simulink model "Hopper_Land_Sim"  (R2023b)
settings: Solver=VariableStepAuto  StartTime=0.0  StopTime=64.5  FixedStep=0.1  MaxStep=0.1  RelTol=1e-6  AbsTol=1e-8
values from neighbouring files (symbols this model uses):
  c_l = 2*sqrt(k_l*m_leg)    [SpringModels.m]
  c_s = 2    [SpringModels.m]
  c_T = 90000    [SpringModels.m]
  C_T = 0.1    [Vehicle_Properties.m]
  g = 1.625    [CalculateLQRGains.m]    (also in IterativeLQR.m; LQR_Controller.m; Trap2D.m = param.g; Vehicle_Properties.m)
  k_l = 100000000000    [SpringModels.m]
  k_s = 500    [SpringModels.m]
  k_T = 9999999    [SpringModels.m]    (also in Vehicle_Properties.m = 0.8)
  K_x = K    [LQR_Controller.m]
  K_y = [K(1), -K(2), K(3), -K(4)]    [LQR_Controller.m]
  l = 4.2926/2    (= 2.1463)    [CalculateLQRGains.m]    (also in IterativeLQR.m; LQR_Controller.m; Vehicle_Properties.m)
  m_e = 150    [CalculateLQRGains.m]    (also in IterativeLQR.m; LQR_Controller.m; Vehicle_Properties.m)
  m_l = 803    [CalculateLQRGains.m]    (also in IterativeLQR.m; LQR_Controller.m; Vehicle_Properties.m)
  m_leg = 10    [SpringModels.m]
  m_s = 355.9/2    (= 177.95)    [SpringModels.m]
  mu_floor = .2    (= 0.2)    [SpringModels.m]
  mu_surface = 0.2    [Vehicle_Properties.m]
  n_floor = [cosd(90+floor_angle), 0, sind(90+floor_angle)]    [FloorModel.m]
  n_surface = [0; 0; 1]    [Vehicle_Properties.m]
  p_l2 = [1; 0; -.5]    [SpringModels.m]
  p_l3 = [0; -1; -.5]    [SpringModels.m]
  p_l4 = [0; 1; -.5]    [SpringModels.m]
  r_l1 = [cosd(angle_legs); 0; sind(leg_length)]    [FloorModel.m]    (also in SpringModels.m = r_l1/norm(r_l1))
  r_l2 = [-cosd(angle_legs); 0; sind(leg_length)]    [FloorModel.m]    (also in SpringModels.m = r_l2/norm(r_l2))
  r_l3 = [0; cosd(angle_legs); sind(leg_length)]    [FloorModel.m]    (also in SpringModels.m = r_l3/norm(r_l3))
  r_l4 = [0; -cosd(angle_legs); sind(leg_length)]    [FloorModel.m]    (also in SpringModels.m = r_l4/norm(r_l4))
libraries: matrix_library x17, slpidlib x5, simulink x2, simulink_extras x1, shared6dof x1, vrlib x1
(part 1 of 2)
settings Model: Creator=Hoboness  LastModifiedBy=tonie

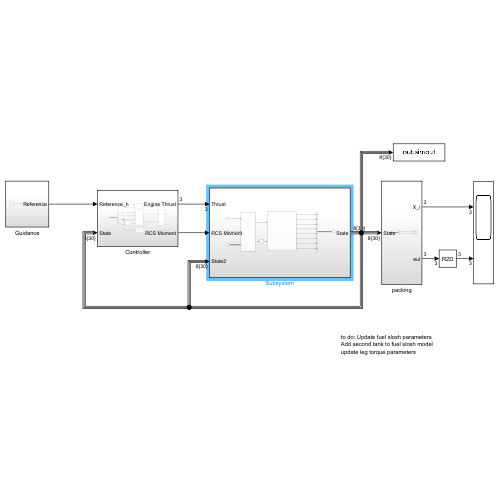
[thumbnail: Simulink's stored preview of the top-level diagram]
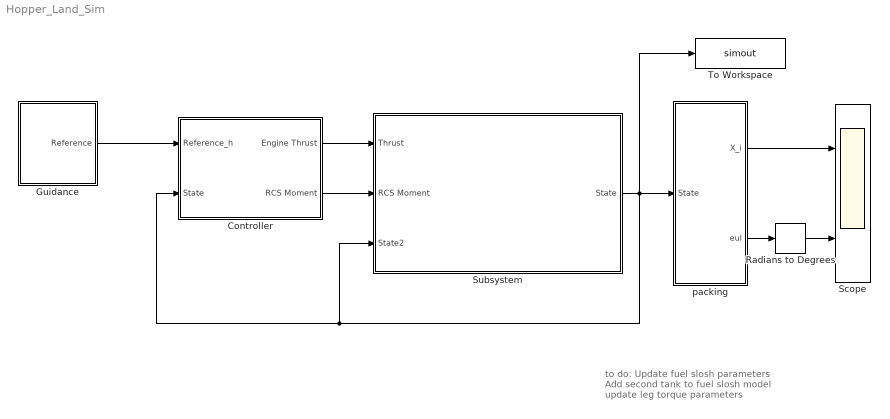
== system Hopper_Land_Sim ==
  note: to do: Update fuel slosh parameters
      | Add second tank to fuel slosh model
      | update leg torque parameters
  Controller : Subsystem
  Guidance : Subsystem
  Radians to Degrees : simulink_extras/Transformations/Radians to Degrees
  Scope : Scope  NumInputPorts=2
  Subsystem : Subsystem
  To Workspace : ToWorkspace  VariableName=simout  SaveFormat=Timeseries  SampleTime=-1
  packing : Subsystem
  wires:
  Subsystem/1(State) -> Subsystem/3(State2), Controller/2(State), packing/1(State), To Workspace/1
  Controller/1(Engine Thrust) -> Subsystem/1(Thrust)
  Guidance/1(Reference) -> Controller/1(Reference_h)
  packing/1(X_i) -> Scope/1
  packing/2(eul) -> Radians to Degrees/1
  Radians to Degrees/1 -> Scope/2
  Controller/2(RCS Moment) -> Subsystem/2(RCS Moment)

== system Hopper_Land_Sim/Controller ==
  Reference_h : Inport
  State : Inport  Port=2
  Bus Selector : BusSelector  OutputSignals=X_i,V_i,euler_a_rad,omega_b
  Psi Control : Subsystem
  Thrust Bounding : Subsystem
  X-Y control : Subsystem
  Z Control : Subsystem
  pqr to theta_dot : Subsystem
  Engine Thrust : Outport
  RCS Moment : Outport  Port=2
  wires:
  Reference_h/1 -> Z Control/1(Reference_h)
  State/1 -> Bus Selector/1
  Bus Selector/1 -> X-Y control/1(<X_i>), Z Control/2(<X_i>)  "<X_i>"
  Bus Selector/2 -> X-Y control/2(V_i)  "<V_i>"
  Bus Selector/4 -> pqr to theta_dot/2(omega_b)  "<omega_b>"
  Bus Selector/3 -> Psi Control/1(euler_a_rad), pqr to theta_dot/1(<euler_a_rad>), X-Y control/3(euler_a_rad)  "<euler_a_rad>"
  Thrust Bounding/1(Thrust) -> Engine Thrust/1
  pqr to theta_dot/1(euler_dot) -> X-Y control/4(euler_dot)
  Psi Control/1(RCS Moment) -> RCS Moment/1
  Z Control/1(Tz) -> Thrust Bounding/1(T_z)
  X-Y control/1(Tx) -> Thrust Bounding/2(Tx)
  X-Y control/2(Ty) -> Thrust Bounding/3(Ty)

== system Hopper_Land_Sim/Guidance ==
  Constant : Constant  Value=14
  Reference : Outport
  wires:
  Constant/1 -> Reference/1

== system Hopper_Land_Sim/Subsystem ==
  Thrust : Inport
  RCS Moment : Inport  Port=2
  State2 : Inport  Port=3
  6DOF (Euler Angles) : shared6dof/6DOF (Euler Angles)  units=Metric (MKS)  mtype=Fixed  rep=Euler Angles  xme_0=[0 0 100]  Vm_0=[0 0 0]  eul_0=deg2rad([0 0 0])  pm_0=[0 0 0]  mass_0=m_e + m_l  mass_e=0.5  mass_f=2.0  inertia=diag([38875.267 39854.689 26895.658]) * 0.3048^2 * 4.44822  inertia_e=eye(3)  inertia_f=2*eye(3)  k_quat=1.0  vre_flag=on  abi_flag=off  aMode=0  xme_statename=''  Vm_statename=''  eul_statename=''  quat_statename=''  pm_statename=''  mass_statename=''
  Bus Creator : BusCreator  Inputs=8
  Calculate Forces and Moments : Subsystem
  Reshape : Reshape
  State : Outport
  wires:
  6DOF (Euler Angles)/3 -> Bus Creator/3  "euler_a_rad"
  6DOF (Euler Angles)/8 -> Bus Creator/8  "A_bb"
  6DOF (Euler Angles)/4 -> Bus Creator/4  "DCM_bi"
  6DOF (Euler Angles)/6 -> Bus Creator/6  "omega_b"
  6DOF (Euler Angles)/7 -> Bus Creator/7  "omega_dot_b"
  6DOF (Euler Angles)/2 -> Bus Creator/2  "X_i"
  Bus Creator/1 -> State/1  "State"
  6DOF (Euler Angles)/1 -> Bus Creator/1  "V_i"
  6DOF (Euler Angles)/5 -> Bus Creator/5  "V_b"
  Thrust/1 -> Calculate Forces and Moments/1(Thrust)
  Calculate Forces and Moments/1(F_b) -> 6DOF (Euler Angles)/1
  Calculate Forces and Moments/2(M_b) -> Reshape/1
  State2/1 -> Calculate Forces and Moments/3(State2)
  RCS Moment/1 -> Calculate Forces and Moments/2(RCS Moment)
  Reshape/1 -> 6DOF (Euler Angles)/2

== system Hopper_Land_Sim/packing ==
  State : Inport
  Bus Selector : BusSelector  OutputSignals=X_i,euler_a_rad
  X_i : Outport
  eul : Outport  Port=2
  wires:
  State/1 -> Bus Selector/1
  Bus Selector/1 -> X_i/1  "<X_i>"
  Bus Selector/2 -> eul/1  "<euler_a_rad>"

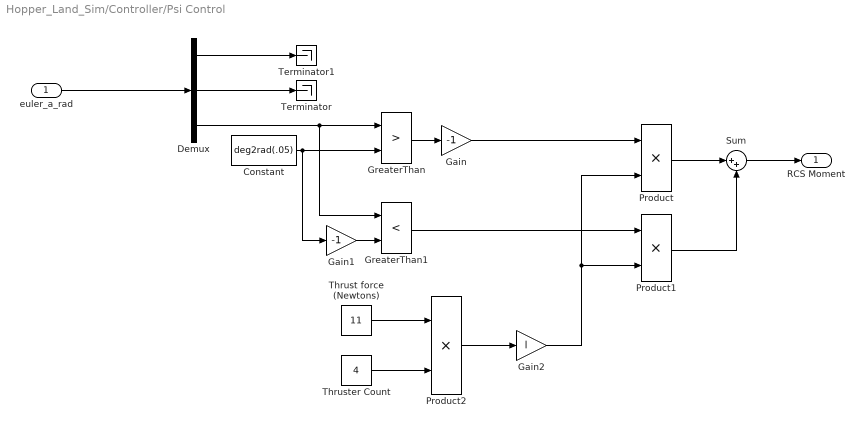
== system Hopper_Land_Sim/Controller/Psi Control ==
  euler_a_rad : Inport
  Constant : Constant  Value=deg2rad(.05)
  Demux : Demux  Outputs=3
  Gain : Gain  Gain=-1
  Gain1 : Gain  Gain=-1
  Gain2 : Gain  Gain=l
  GreaterThan : RelationalOperator  Operator=>  OutDataTypeStr=boolean  RndMeth=Simplest  InputSameDT=off
  GreaterThan1 : RelationalOperator  Operator=<  OutDataTypeStr=boolean  RndMeth=Simplest  InputSameDT=off
  Product : Product
  Product1 : Product
  Product2 : Product
  Sum : Sum  Inputs=|++
  Terminator : Terminator
  Terminator1 : Terminator
  Thrust force (Newtons) : Constant  Value=11
  Thruster Count : Constant  Value=4
  RCS Moment : Outport
  wires:
  euler_a_rad/1 -> Demux/1
  Demux/3 -> GreaterThan1/1, GreaterThan/1
  Demux/2 -> Terminator/1
  Demux/1 -> Terminator1/1
  Constant/1 -> GreaterThan/2, Gain1/1
  GreaterThan/1 -> Gain/1
  Gain/1 -> Product/1
  Product/1 -> Sum/1
  Gain1/1 -> GreaterThan1/2
  GreaterThan1/1 -> Product1/1
  Product1/1 -> Sum/2
  Thrust force (Newtons)/1 -> Product2/1
  Thruster Count/1 -> Product2/2
  Product2/1 -> Gain2/1
  Sum/1 -> RCS Moment/1
  Gain2/1 -> Product/2, Product1/2

== system Hopper_Land_Sim/Controller/Thrust Bounding ==
  T_z : Inport
  Tx : Inport  Port=2
  Ty : Inport  Port=3
  Vector Concatenate : Concatenate  NumInputs=3
  Thrust : Outport
  wires:
  T_z/1 -> Vector Concatenate/3
  Vector Concatenate/1 -> Thrust/1
  Ty/1 -> Vector Concatenate/2
  Tx/1 -> Vector Concatenate/1

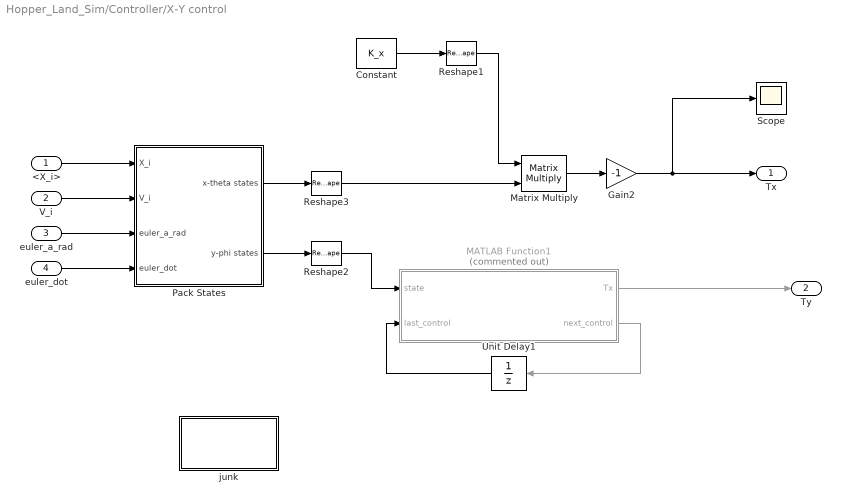
== system Hopper_Land_Sim/Controller/X-Y control ==
  <X_i> : Inport
  V_i : Inport  Port=2
  euler_a_rad : Inport  Port=3
  euler_dot : Inport  Port=4
  Constant : Constant  Value=K_x
  Gain2 : Gain  Gain=-1
  MATLAB Function1 : MATLAB Function  Commented=on  TreatAsAtomicUnit=on
  Matrix Multiply : Product  Multiplication=Matrix(*)
  "Pack States " : Subsystem
  Reshape1 : Reshape  OutputDimensionality=Row vector (2-D)
  Reshape2 : Reshape  OutputDimensionality=Column vector (2-D)
  Reshape3 : Reshape  OutputDimensionality=Column vector (2-D)
  Scope : Scope
  Unit Delay1 : UnitDelay  SampleTime=-1  HasFrameUpgradeWarning=on
  junk : Subsystem
  Tx : Outport
  Ty : Outport  Port=2
  wires:
  <X_i>/1 -> "Pack States "/1(X_i)
  V_i/1 -> "Pack States "/2(V_i)
  euler_a_rad/1 -> "Pack States "/3(euler_a_rad)
  euler_dot/1 -> "Pack States "/4(euler_dot)
  "Pack States "/2(y-phi states) -> Reshape2/1
  "Pack States "/1(x-theta states) -> Reshape3/1
  MATLAB Function1/1(Tx) -> Ty/1
  MATLAB Function1/2(next_control) -> Unit Delay1/1
  Unit Delay1/1 -> MATLAB Function1/2(last_control)
  Reshape2/1 -> MATLAB Function1/1(state)
  Gain2/1 -> Scope/1, Tx/1
  Constant/1 -> Reshape1/1
  Matrix Multiply/1 -> Gain2/1
  Reshape1/1 -> Matrix Multiply/1
  Reshape3/1 -> Matrix Multiply/2

== system Hopper_Land_Sim/Controller/Z Control ==
  Reference_h : Inport
  <X_i> : Inport  Port=2
  PID Controller : slpidlib/PID Controller  Controller=PID  Form=Parallel  TimeDomain=Continuous-time  UseExternalTs=off  SampleTime=-1  IntegratorMethod=Forward Euler  FilterMethod=Forward Euler  ControllerParametersSource=internal  P=522.596849697367  I=13.9356720912904  UseKiTs=off  D=12000  N=1  UseFilter=on  TunerSelectOption=Transfer Function Based (PID Tuner App)  InitialConditionSource=internal  InitialConditionForIntegrator=100  InitialConditionForFilter=100  DifferentiatorICPrevScaledInput=0  ExternalReset=none  TrackingMode=off  Kt=1  LimitOutput=on  SatLimitsSource=internal  UpperSaturationLimit=24000  LowerSaturationLimit=100  LinearizeAsGain=on  AntiWindupMode=none  Kb=1  LimitIntegrator=off  UpperIntegratorSaturationLimit=inf  LowerIntegratorSaturationLimit=-inf  POutMin=[]  POutMax=[]  IOutMin=[]  IOutMax=[]  DOutMin=[]  DOutMax=[]  NOutMin=[]  NOutMax=[]  SumOutMin=[]  SumOutMax=[]  SaturationOutMin=[]  SaturationOutMax=[]  PParamMin=[]  PParamMax=[]  IParamMin=[]  IParamMax=[]  DParamMin=[]  DParamMax=[]  NParamMin=[]  NParamMax=[]  KbParamMin=[]  KbParamMax=[]  KtParamMin=[]  KtParamMax=[]  KbOutMin=[]  KbOutMax=[]  KtOutMin=[]  KtOutMax=[]  IntegratorOutMin=[]  IntegratorOutMax=[]  FilterOutMin=[]  FilterOutMax=[]  SumI1OutMin=[]  SumI1OutMax=[]  SumI2OutMin=[]  SumI2OutMax=[]  SumI3OutMin=[]  SumI3OutMax=[]  SumI4OutMin=[]  SumI4OutMax=[]  SumDOutMin=[]  SumDOutMax=[]  DifferentiatorOutMin=[]  DifferentiatorOutMax=[]  FilterDiffOutCoefMin=[]  FilterDiffOutCoefMax=[]  ReciprocalOutMin=[]  ReciprocalOutMax=[]  SumDenOutMin=[]  SumDenOutMax=[]  SumNumOutMin=[]  SumNumOutMax=[]  DivideOutMin=[]  DivideOutMax=[]  UdiffTsProdOutMin=[]  UdiffTsProdOutMax=[]  NTsProdOutMin=[]  NTsProdOutMax=[]  UintegralTsProdOutMin=[]  UintegralTsProdOutMax=[]  UngainTsProdOutMin=[]  UngainTsProdOutMax=[]  ClampingZeroOutDataTypeStr=Inherit: Inherit via back propagation  ClampingZeroOutMin=[]  ClampingZeroOutMax=[]  FilterDenConstantOutDataTypeStr=Inherit: Inherit via back propagation  FilterDenConstantOutMin=[]  FilterDenConstantOutMax=[]  PCopyOutDataTypeStr=Inherit: Inherit via back propagation  PCopyOutMin=[]  PCopyOutMax=[]  NCopyOutDataTypeStr=Inherit: Inherit via back propagation  NCopyOutMin=[]  NCopyOutMax=[]  IntegratorContinuousStateAttributes=''  IntegratorStateMustResolveToSignalObject=off  IntegratorRTWStateStorageClass=Auto  FilterContinuousStateAttributes=''  FilterStateMustResolveToSignalObject=off  FilterRTWStateStorageClass=Auto  ParallelPVariant=InternalParameters  IdealPVariant=Disabled  IVariant=InternalParameters  DVariant=InternalParameters  IntegratorVariant=Continuous  SatVariant=Enabled  AWVariant=Passthrough  PCopyVariant=Disabled  TRVariant=Disabled  FdbkBlocksVariant=Forward  IdealPFdbkVariant=Disabled  SatFdbkVariant=Disabled  DerivativeFilterVariant=ContFilter  NVariant=InternalParameters  NCopyVariant=Disabled  FilterICVariant=InternalICsFilter  IntegratorICVariant=InternalICs  ExternalResetVariant=Disabled  TRSumVariant=Passthrough  SumFdbkVariant=Disabled  SumVariant=Sum_PID  TsampFilterVariant=InternalTs  TsampNgainVariant=Passthrough  TsampIntegralVariant=Disabled_SignalSpec  ExternalSaturationOutDataTypeStr=Inherit: Same as second input
  Selector : Selector  InputPortWidth=3  IndexOptions=Index vector (dialog)  Indices=3  OutputSizes=1
  Sum : Sum  Inputs=+-|
  Tz : Outport
  wires:
  Reference_h/1 -> Sum/1
  Sum/1 -> PID Controller/1
  Selector/1 -> Sum/2  "alt_m"
  PID Controller/1 -> Tz/1  "T_z"
  <X_i>/1 -> Selector/1

== system Hopper_Land_Sim/Controller/pqr to theta_dot ==
  <euler_a_rad> : Inport
  omega_b : Inport  Port=2
  MATLAB Function : MATLAB Function  TreatAsAtomicUnit=on
  euler_dot : Outport
  wires:
  omega_b/1 -> MATLAB Function/2(omega_b)
  <euler_a_rad>/1 -> MATLAB Function/1(euler_a_rad)
  MATLAB Function/1(euler_dot) -> euler_dot/1

== system Hopper_Land_Sim/Subsystem/Calculate Forces and Moments ==
  Thrust : Inport
  RCS Moment : Inport  Port=2
  State2 : Inport  Port=3
  Disturbances : Subsystem
  Ground : Subsystem
  Sum Forces : Subsystem
  Sum Moments : Subsystem
  F_b : Outport
  M_b : Outport  Port=2
  wires:
  Thrust/1 -> Disturbances/1(Thurst), Sum Moments/1(Thrust), Sum Forces/1(Thrust)
  State2/1 -> Ground/1(State2), Sum Forces/3(state)
  Sum Forces/1(Force_out) -> F_b/1
  Sum Moments/1(M_b) -> M_b/1
  RCS Moment/1 -> Sum Moments/2(RCS Moment)
  Disturbances/1(Disturbance Force) -> Sum Forces/2(Disturbance Forces)
  Disturbances/2(Disturbance Moment) -> Sum Moments/3(Disturbance Moments)
  Ground/1(Ground Force) -> Sum Forces/4(Ground Force)
  Ground/2(Ground Moments) -> Sum Moments/4(Ground Moments)

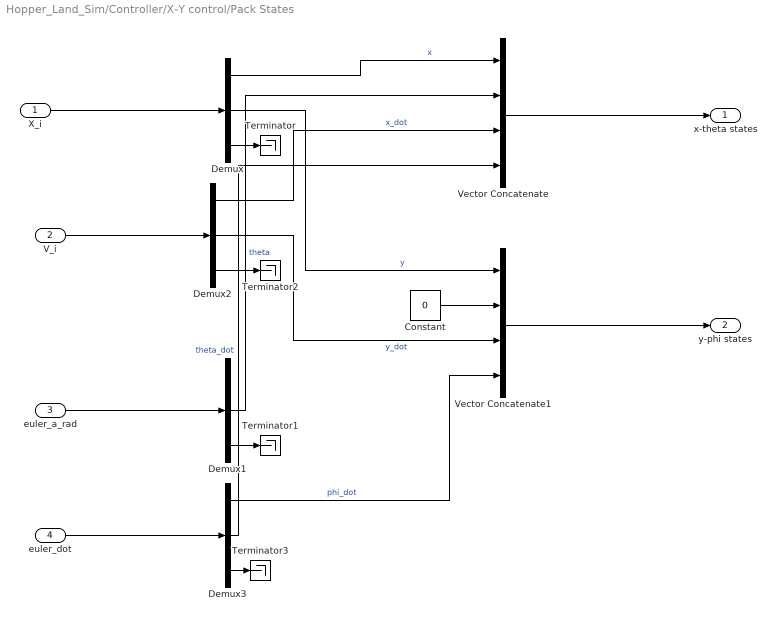
== system Hopper_Land_Sim/Controller/X-Y control/Pack States  ==
  X_i : Inport
  V_i : Inport  Port=2
  euler_a_rad : Inport  Port=3
  euler_dot : Inport  Port=4
  Constant : Constant  Value=0
  Demux{,1..3} (4 alike) : Demux  Outputs=3
  Terminator{,1..3} (4 alike) : Terminator
  Vector Concatenate : Concatenate  NumInputs=4
  Vector Concatenate1 : Concatenate  NumInputs=4
  x-theta states : Outport
  y-phi states : Outport  Port=2
  wires:
  Demux2/2 -> Vector Concatenate1/3  "y_dot"
  Demux/1 -> Vector Concatenate/1  "x"
  Demux2/1 -> Vector Concatenate/3  "x_dot"
  V_i/1 -> Demux2/1
  Demux1/3 -> Terminator1/1
  Demux/2 -> Vector Concatenate1/1  "y"
  Demux2/3 -> Terminator2/1
  Demux/3 -> Terminator/1
  Demux3/3 -> Terminator3/1
  Vector Concatenate/1 -> x-theta states/1
  X_i/1 -> Demux/1
  euler_a_rad/1 -> Demux1/1
  euler_dot/1 -> Demux3/1
  Vector Concatenate1/1 -> y-phi states/1
  Demux3/1 -> Vector Concatenate1/4  "phi_dot"
  Demux1/2 -> Vector Concatenate/2  "theta"
  Demux3/2 -> Vector Concatenate/4  "theta_dot"
  Constant/1 -> Vector Concatenate1/2

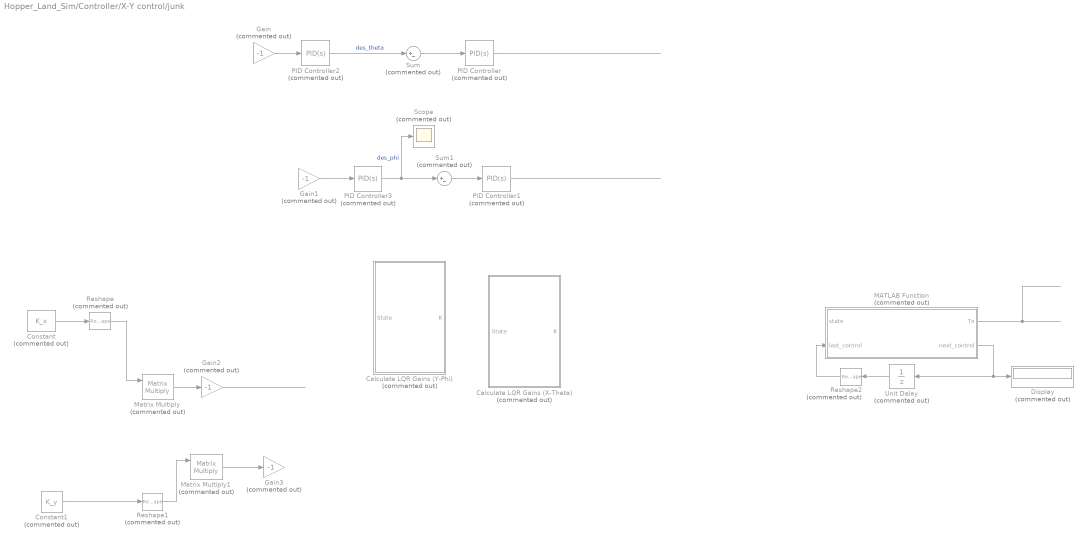
== system Hopper_Land_Sim/Controller/X-Y control/junk ==
  Calculate LQR Gains (X-Theta) : MATLAB Function  Commented=on  TreatAsAtomicUnit=on  SystemSampleTime=9999999999999
  Calculate LQR Gains (Y-Phi) : MATLAB Function  Commented=on  TreatAsAtomicUnit=on  SystemSampleTime=9999999999999
  Constant : Constant  Commented=on  Value=K_x
  Constant1 : Constant  Commented=on  Value=K_y
  Display : Display  Commented=on
  Gain{,1..3} (4 alike) : Gain  Commented=on  Gain=-1
  MATLAB Function : MATLAB Function  Commented=on  TreatAsAtomicUnit=on
  Matrix Multiply : Product  Commented=on  Multiplication=Matrix(*)
  Matrix Multiply1 : Product  Commented=on  Multiplication=Matrix(*)
  PID Controller : slpidlib/PID Controller  Commented=on  Controller=PID  Form=Parallel  TimeDomain=Continuous-time  UseExternalTs=off  SampleTime=-1  IntegratorMethod=Forward Euler  FilterMethod=Forward Euler  ControllerParametersSource=internal  P=43430.8852214789  I=11554.268575592  UseKiTs=off  D=39980.5566743985  N=32.1920872149426  UseFilter=on  TunerSelectOption=Transfer Function Based (PID Tuner App)  InitialConditionSource=internal  InitialConditionForIntegrator=0  InitialConditionForFilter=0  DifferentiatorICPrevScaledInput=0  ExternalReset=none  TrackingMode=off  Kt=1  LimitOutput=off  SatLimitsSource=internal  UpperSaturationLimit=inf  LowerSaturationLimit=-inf  LinearizeAsGain=on  AntiWindupMode=none  Kb=1  LimitIntegrator=off  UpperIntegratorSaturationLimit=inf  LowerIntegratorSaturationLimit=-inf  POutMin=[]  POutMax=[]  IOutMin=[]  IOutMax=[]  DOutMin=[]  DOutMax=[]  NOutMin=[]  NOutMax=[]  SumOutMin=[]  SumOutMax=[]  SaturationOutMin=[]  SaturationOutMax=[]  PParamMin=[]  PParamMax=[]  IParamMin=[]  IParamMax=[]  DParamMin=[]  DParamMax=[]  NParamMin=[]  NParamMax=[]  KbParamMin=[]  KbParamMax=[]  KtParamMin=[]  KtParamMax=[]  KbOutMin=[]  KbOutMax=[]  KtOutMin=[]  KtOutMax=[]  IntegratorOutMin=[]  IntegratorOutMax=[]  FilterOutMin=[]  FilterOutMax=[]  SumI1OutMin=[]  SumI1OutMax=[]  SumI2OutMin=[]  SumI2OutMax=[]  SumI3OutMin=[]  SumI3OutMax=[]  SumI4OutMin=[]  SumI4OutMax=[]  SumDOutMin=[]  SumDOutMax=[]  DifferentiatorOutMin=[]  DifferentiatorOutMax=[]  FilterDiffOutCoefMin=[]  FilterDiffOutCoefMax=[]  ReciprocalOutMin=[]  ReciprocalOutMax=[]  SumDenOutMin=[]  SumDenOutMax=[]  SumNumOutMin=[]  SumNumOutMax=[]  DivideOutMin=[]  DivideOutMax=[]  UdiffTsProdOutMin=[]  UdiffTsProdOutMax=[]  NTsProdOutMin=[]  NTsProdOutMax=[]  UintegralTsProdOutMin=[]  UintegralTsProdOutMax=[]  UngainTsProdOutMin=[]  UngainTsProdOutMax=[]  ClampingZeroOutDataTypeStr=Inherit: Inherit via back propagation  ClampingZeroOutMin=[]  ClampingZeroOutMax=[]  FilterDenConstantOutDataTypeStr=Inherit: Inherit via back propagation  FilterDenConstantOutMin=[]  FilterDenConstantOutMax=[]  PCopyOutDataTypeStr=Inherit: Inherit via back propagation  PCopyOutMin=[]  PCopyOutMax=[]  NCopyOutDataTypeStr=Inherit: Inherit via back propagation  NCopyOutMin=[]  NCopyOutMax=[]  IntegratorContinuousStateAttributes=''  IntegratorStateMustResolveToSignalObject=off  IntegratorRTWStateStorageClass=Auto  FilterContinuousStateAttributes=''  FilterStateMustResolveToSignalObject=off  FilterRTWStateStorageClass=Auto  ParallelPVariant=InternalParameters  IdealPVariant=Disabled  IVariant=InternalParameters  DVariant=InternalParameters  IntegratorVariant=Continuous  SatVariant=Disabled  AWVariant=Passthrough  PCopyVariant=Disabled  TRVariant=Disabled  FdbkBlocksVariant=Forward  IdealPFdbkVariant=Disabled  SatFdbkVariant=Disabled  DerivativeFilterVariant=ContFilter  NVariant=InternalParameters  NCopyVariant=Disabled  FilterICVariant=InternalICsFilter  IntegratorICVariant=InternalICs  ExternalResetVariant=Disabled  TRSumVariant=Passthrough  SumFdbkVariant=Disabled  SumVariant=Sum_PID  TsampFilterVariant=InternalTs  TsampNgainVariant=Passthrough  TsampIntegralVariant=Disabled_SignalSpec  ExternalSaturationOutDataTypeStr=Inherit: Same as second input
  PID Controller1 : slpidlib/PID Controller  Commented=on  Controller=PID  Form=Parallel  TimeDomain=Continuous-time  UseExternalTs=off  SampleTime=-1  IntegratorMethod=Forward Euler  FilterMethod=Forward Euler  ControllerParametersSource=internal  P=43430.8852214789  I=11554.268575592  UseKiTs=off  D=39980.5566743985  N=32.1920872149426  UseFilter=on  TunerSelectOption=Transfer Function Based (PID Tuner App)  InitialConditionSource=internal  InitialConditionForIntegrator=0  InitialConditionForFilter=0  DifferentiatorICPrevScaledInput=0  ExternalReset=none  TrackingMode=off  Kt=1  LimitOutput=off  SatLimitsSource=internal  UpperSaturationLimit=inf  LowerSaturationLimit=-inf  LinearizeAsGain=on  AntiWindupMode=none  Kb=1  LimitIntegrator=off  UpperIntegratorSaturationLimit=inf  LowerIntegratorSaturationLimit=-inf  POutMin=[]  POutMax=[]  IOutMin=[]  IOutMax=[]  DOutMin=[]  DOutMax=[]  NOutMin=[]  NOutMax=[]  SumOutMin=[]  SumOutMax=[]  SaturationOutMin=[]  SaturationOutMax=[]  PParamMin=[]  PParamMax=[]  IParamMin=[]  IParamMax=[]  DParamMin=[]  DParamMax=[]  NParamMin=[]  NParamMax=[]  KbParamMin=[]  KbParamMax=[]  KtParamMin=[]  KtParamMax=[]  KbOutMin=[]  KbOutMax=[]  KtOutMin=[]  KtOutMax=[]  IntegratorOutMin=[]  IntegratorOutMax=[]  FilterOutMin=[]  FilterOutMax=[]  SumI1OutMin=[]  SumI1OutMax=[]  SumI2OutMin=[]  SumI2OutMax=[]  SumI3OutMin=[]  SumI3OutMax=[]  SumI4OutMin=[]  SumI4OutMax=[]  SumDOutMin=[]  SumDOutMax=[]  DifferentiatorOutMin=[]  DifferentiatorOutMax=[]  FilterDiffOutCoefMin=[]  FilterDiffOutCoefMax=[]  ReciprocalOutMin=[]  ReciprocalOutMax=[]  SumDenOutMin=[]  SumDenOutMax=[]  SumNumOutMin=[]  SumNumOutMax=[]  DivideOutMin=[]  DivideOutMax=[]  UdiffTsProdOutMin=[]  UdiffTsProdOutMax=[]  NTsProdOutMin=[]  NTsProdOutMax=[]  UintegralTsProdOutMin=[]  UintegralTsProdOutMax=[]  UngainTsProdOutMin=[]  UngainTsProdOutMax=[]  ClampingZeroOutDataTypeStr=Inherit: Inherit via back propagation  ClampingZeroOutMin=[]  ClampingZeroOutMax=[]  FilterDenConstantOutDataTypeStr=Inherit: Inherit via back propagation  FilterDenConstantOutMin=[]  FilterDenConstantOutMax=[]  PCopyOutDataTypeStr=Inherit: Inherit via back propagation  PCopyOutMin=[]  PCopyOutMax=[]  NCopyOutDataTypeStr=Inherit: Inherit via back propagation  NCopyOutMin=[]  NCopyOutMax=[]  IntegratorContinuousStateAttributes=''  IntegratorStateMustResolveToSignalObject=off  IntegratorRTWStateStorageClass=Auto  FilterContinuousStateAttributes=''  FilterStateMustResolveToSignalObject=off  FilterRTWStateStorageClass=Auto  ParallelPVariant=InternalParameters  IdealPVariant=Disabled  IVariant=InternalParameters  DVariant=InternalParameters  IntegratorVariant=Continuous  SatVariant=Disabled  AWVariant=Passthrough  PCopyVariant=Disabled  TRVariant=Disabled  FdbkBlocksVariant=Forward  IdealPFdbkVariant=Disabled  SatFdbkVariant=Disabled  DerivativeFilterVariant=ContFilter  NVariant=InternalParameters  NCopyVariant=Disabled  FilterICVariant=InternalICsFilter  IntegratorICVariant=InternalICs  ExternalResetVariant=Disabled  TRSumVariant=Passthrough  SumFdbkVariant=Disabled  SumVariant=Sum_PID  TsampFilterVariant=InternalTs  TsampNgainVariant=Passthrough  TsampIntegralVariant=Disabled_SignalSpec  ExternalSaturationOutDataTypeStr=Inherit: Same as second input
  PID Controller2 : slpidlib/PID Controller  Commented=on  Controller=PID  Form=Parallel  TimeDomain=Continuous-time  UseExternalTs=off  SampleTime=-1  IntegratorMethod=Forward Euler  FilterMethod=Forward Euler  ControllerParametersSource=internal  P=0.0149555658055821  I=0.00505656866824881  UseKiTs=off  D=0  N=100  UseFilter=on  TunerSelectOption=Transfer Function Based (PID Tuner App)  InitialConditionSource=internal  InitialConditionForIntegrator=0  InitialConditionForFilter=0  DifferentiatorICPrevScaledInput=0  ExternalReset=none  TrackingMode=off  Kt=1  LimitOutput=off  SatLimitsSource=internal  UpperSaturationLimit=inf  LowerSaturationLimit=-inf  LinearizeAsGain=on  AntiWindupMode=none  Kb=1  LimitIntegrator=off  UpperIntegratorSaturationLimit=inf  LowerIntegratorSaturationLimit=-inf  POutMin=[]  POutMax=[]  IOutMin=[]  IOutMax=[]  DOutMin=[]  DOutMax=[]  NOutMin=[]  NOutMax=[]  SumOutMin=[]  SumOutMax=[]  SaturationOutMin=[]  SaturationOutMax=[]  PParamMin=[]  PParamMax=[]  IParamMin=[]  IParamMax=[]  DParamMin=[]  DParamMax=[]  NParamMin=[]  NParamMax=[]  KbParamMin=[]  KbParamMax=[]  KtParamMin=[]  KtParamMax=[]  KbOutMin=[]  KbOutMax=[]  KtOutMin=[]  KtOutMax=[]  IntegratorOutMin=[]  IntegratorOutMax=[]  FilterOutMin=[]  FilterOutMax=[]  SumI1OutMin=[]  SumI1OutMax=[]  SumI2OutMin=[]  SumI2OutMax=[]  SumI3OutMin=[]  SumI3OutMax=[]  SumI4OutMin=[]  SumI4OutMax=[]  SumDOutMin=[]  SumDOutMax=[]  DifferentiatorOutMin=[]  DifferentiatorOutMax=[]  FilterDiffOutCoefMin=[]  FilterDiffOutCoefMax=[]  ReciprocalOutMin=[]  ReciprocalOutMax=[]  SumDenOutMin=[]  SumDenOutMax=[]  SumNumOutMin=[]  SumNumOutMax=[]  DivideOutMin=[]  DivideOutMax=[]  UdiffTsProdOutMin=[]  UdiffTsProdOutMax=[]  NTsProdOutMin=[]  NTsProdOutMax=[]  UintegralTsProdOutMin=[]  UintegralTsProdOutMax=[]  UngainTsProdOutMin=[]  UngainTsProdOutMax=[]  ClampingZeroOutDataTypeStr=Inherit: Inherit via back propagation  ClampingZeroOutMin=[]  ClampingZeroOutMax=[]  FilterDenConstantOutDataTypeStr=Inherit: Inherit via back propagation  FilterDenConstantOutMin=[]  FilterDenConstantOutMax=[]  PCopyOutDataTypeStr=Inherit: Inherit via back propagation  PCopyOutMin=[]  PCopyOutMax=[]  NCopyOutDataTypeStr=Inherit: Inherit via back propagation  NCopyOutMin=[]  NCopyOutMax=[]  IntegratorContinuousStateAttributes=''  IntegratorStateMustResolveToSignalObject=off  IntegratorRTWStateStorageClass=Auto  FilterContinuousStateAttributes=''  FilterStateMustResolveToSignalObject=off  FilterRTWStateStorageClass=Auto  ParallelPVariant=InternalParameters  IdealPVariant=Disabled  IVariant=InternalParameters  DVariant=InternalParameters  IntegratorVariant=Continuous  SatVariant=Disabled  AWVariant=Passthrough  PCopyVariant=Disabled  TRVariant=Disabled  FdbkBlocksVariant=Forward  IdealPFdbkVariant=Disabled  SatFdbkVariant=Disabled  DerivativeFilterVariant=ContFilter  NVariant=InternalParameters  NCopyVariant=Disabled  FilterICVariant=InternalICsFilter  IntegratorICVariant=InternalICs  ExternalResetVariant=Disabled  TRSumVariant=Passthrough  SumFdbkVariant=Disabled  SumVariant=Sum_PID  TsampFilterVariant=InternalTs  TsampNgainVariant=Passthrough  TsampIntegralVariant=Disabled_SignalSpec  ExternalSaturationOutDataTypeStr=Inherit: Same as second input
  PID Controller3 : slpidlib/PID Controller  Commented=on  Controller=PID  Form=Parallel  TimeDomain=Continuous-time  UseExternalTs=off  SampleTime=-1  IntegratorMethod=Forward Euler  FilterMethod=Forward Euler  ControllerParametersSource=internal  P=0.0149555658055821  I=0.00505656866824881  UseKiTs=off  D=0  N=100  UseFilter=on  TunerSelectOption=Transfer Function Based (PID Tuner App)  InitialConditionSource=internal  InitialConditionForIntegrator=0  InitialConditionForFilter=0  DifferentiatorICPrevScaledInput=0  ExternalReset=none  TrackingMode=off  Kt=1  LimitOutput=off  SatLimitsSource=internal  UpperSaturationLimit=inf  LowerSaturationLimit=-inf  LinearizeAsGain=on  AntiWindupMode=none  Kb=1  LimitIntegrator=off  UpperIntegratorSaturationLimit=inf  LowerIntegratorSaturationLimit=-inf  POutMin=[]  POutMax=[]  IOutMin=[]  IOutMax=[]  DOutMin=[]  DOutMax=[]  NOutMin=[]  NOutMax=[]  SumOutMin=[]  SumOutMax=[]  SaturationOutMin=[]  SaturationOutMax=[]  PParamMin=[]  PParamMax=[]  IParamMin=[]  IParamMax=[]  DParamMin=[]  DParamMax=[]  NParamMin=[]  NParamMax=[]  KbParamMin=[]  KbParamMax=[]  KtParamMin=[]  KtParamMax=[]  KbOutMin=[]  KbOutMax=[]  KtOutMin=[]  KtOutMax=[]  IntegratorOutMin=[]  IntegratorOutMax=[]  FilterOutMin=[]  FilterOutMax=[]  SumI1OutMin=[]  SumI1OutMax=[]  SumI2OutMin=[]  SumI2OutMax=[]  SumI3OutMin=[]  SumI3OutMax=[]  SumI4OutMin=[]  SumI4OutMax=[]  SumDOutMin=[]  SumDOutMax=[]  DifferentiatorOutMin=[]  DifferentiatorOutMax=[]  FilterDiffOutCoefMin=[]  FilterDiffOutCoefMax=[]  ReciprocalOutMin=[]  ReciprocalOutMax=[]  SumDenOutMin=[]  SumDenOutMax=[]  SumNumOutMin=[]  SumNumOutMax=[]  DivideOutMin=[]  DivideOutMax=[]  UdiffTsProdOutMin=[]  UdiffTsProdOutMax=[]  NTsProdOutMin=[]  NTsProdOutMax=[]  UintegralTsProdOutMin=[]  UintegralTsProdOutMax=[]  UngainTsProdOutMin=[]  UngainTsProdOutMax=[]  ClampingZeroOutDataTypeStr=Inherit: Inherit via back propagation  ClampingZeroOutMin=[]  ClampingZeroOutMax=[]  FilterDenConstantOutDataTypeStr=Inherit: Inherit via back propagation  FilterDenConstantOutMin=[]  FilterDenConstantOutMax=[]  PCopyOutDataTypeStr=Inherit: Inherit via back propagation  PCopyOutMin=[]  PCopyOutMax=[]  NCopyOutDataTypeStr=Inherit: Inherit via back propagation  NCopyOutMin=[]  NCopyOutMax=[]  IntegratorContinuousStateAttributes=''  IntegratorStateMustResolveToSignalObject=off  IntegratorRTWStateStorageClass=Auto  FilterContinuousStateAttributes=''  FilterStateMustResolveToSignalObject=off  FilterRTWStateStorageClass=Auto  ParallelPVariant=InternalParameters  IdealPVariant=Disabled  IVariant=InternalParameters  DVariant=InternalParameters  IntegratorVariant=Continuous  SatVariant=Disabled  AWVariant=Passthrough  PCopyVariant=Disabled  TRVariant=Disabled  FdbkBlocksVariant=Forward  IdealPFdbkVariant=Disabled  SatFdbkVariant=Disabled  DerivativeFilterVariant=ContFilter  NVariant=InternalParameters  NCopyVariant=Disabled  FilterICVariant=InternalICsFilter  IntegratorICVariant=InternalICs  ExternalResetVariant=Disabled  TRSumVariant=Passthrough  SumFdbkVariant=Disabled  SumVariant=Sum_PID  TsampFilterVariant=InternalTs  TsampNgainVariant=Passthrough  TsampIntegralVariant=Disabled_SignalSpec  ExternalSaturationOutDataTypeStr=Inherit: Same as second input
  Reshape : Reshape  Commented=on  OutputDimensionality=Row vector (2-D)
  Reshape1 : Reshape  Commented=on  OutputDimensionality=Row vector (2-D)
  Reshape2 : Reshape  Commented=on  OutputDimensionality=Row vector (2-D)
  Scope : Scope  Commented=on
  Sum : Sum  Commented=on  Inputs=|+-
  Sum1 : Sum  Commented=on  Inputs=|+-
  Unit Delay : UnitDelay  Commented=on  InitialCondition=zeros(1,80)  SampleTime=-1  HasFrameUpgradeWarning=on
  wires:
  PID Controller3/1 -> Scope/1, Sum1/1  "des_phi"
  PID Controller1/1 -> ?
  ? -> Gain/1  "X"
  ? -> Sum1/2
  ? -> Gain1/1
  Gain1/1 -> PID Controller3/1
  PID Controller2/1 -> Sum/1  "des_theta"
  PID Controller/1 -> ?
  Sum1/1 -> PID Controller1/1
  Sum/1 -> PID Controller/1
  ? -> Sum/2
  Gain/1 -> PID Controller2/1
  Gain2/1 -> ?
  Matrix Multiply/1 -> Gain2/1
  Matrix Multiply1/1 -> Gain3/1
  Constant/1 -> Reshape/1
  Reshape1/1 -> Matrix Multiply1/1
  Constant1/1 -> Reshape1/1
  ? -> ?
  ? -> ?
  Reshape/1 -> Matrix Multiply/1
  Reshape2/1 -> MATLAB Function/2(last_control)
  MATLAB Function/1(Tx) -> ?
  ? -> MATLAB Function/1(state)
  Unit Delay/1 -> Reshape2/1
  MATLAB Function/2(next_control) -> Display/1, Unit Delay/1

== system Hopper_Land_Sim/Subsystem/Calculate Forces and Moments/Disturbances ==
  Thurst : Inport
  Fuel Slosh : Subsystem
  Disturbance Force : Outport
  Disturbance Moment : Outport  Port=2
  wires:
  Thurst/1 -> Fuel Slosh/1(Thrust)
  Fuel Slosh/1(Disturbance Force) -> Disturbance Force/1
  Fuel Slosh/2(Disturbance Moment) -> Disturbance Moment/1

== system Hopper_Land_Sim/Subsystem/Calculate Forces and Moments/Ground ==
  State2 : Inport
  Floor Model : Subsystem
  Floor Model1 : Subsystem  Commented=on
  Leg Model : Subsystem
  Ground Force : Outport
  Ground Moments : Outport  Port=2
  wires:
  State2/1 -> Floor Model1/1(In1), Floor Model/1(In1)
  Floor Model/1(f_T) -> Leg Model/1(f_T)
  Leg Model/1(Leg Force) -> ?
  Leg Model/2(Leg Moment) -> ?
  Floor Model1/1(f_T) -> ?

== system Hopper_Land_Sim/Subsystem/Calculate Forces and Moments/Sum Forces ==
  Thrust : Inport
  Disturbance Forces : Inport  Port=2
  state : Inport  Port=3
  Ground Force : Inport  Port=4
  Add : Sum  Inputs=++++
  Fake ground : Subsystem  Commented=on
  Gravity : Subsystem
  Ground : Subsystem  Commented=on
  Force_out : Outport
  wires:
  Gravity/1(gravity) -> Add/4
  state/1 -> Gravity/1(state), Fake ground/2(state)
  Disturbance Forces/1 -> Add/2
  Add/1 -> Force_out/1
  Thrust/1 -> Add/1
  Ground Force/1 -> Add/3

== system Hopper_Land_Sim/Subsystem/Calculate Forces and Moments/Sum Moments ==
  Thrust : Inport
  RCS Moment : Inport  Port=2
  Disturbance Moments : Inport  Port=3
  Ground Moments : Inport  Port=4
  Add : Sum  Inputs=++++
  Constant : Constant  Value=[0; 0; l]
  Constant1 : Constant  Value=0
  Cross Product : matrix_library/Cross Product
  Reshape : Reshape  OutputDimensionality=Column vector (2-D)
  Reshape1 : Reshape  OutputDimensionality=Column vector (2-D)
  Vector Concatenate : Concatenate  NumInputs=3
  M_b : Outport
  wires:
  Cross Product/1 -> Reshape/1
  Thrust/1 -> Cross Product/2
  Disturbance Moments/1 -> Add/3
  Constant/1 -> Cross Product/1
  Constant1/1 -> Vector Concatenate/2, Vector Concatenate/1
  RCS Moment/1 -> Vector Concatenate/3
  Vector Concatenate/1 -> Reshape1/1
  Reshape/1 -> Add/1
  Reshape1/1 -> Add/2
  Ground Moments/1 -> Add/4
  Add/1 -> M_b/1

== system Hopper_Land_Sim/Subsystem/Calculate Forces and Moments/Disturbances/Fuel Slosh ==
  Thrust : Inport
  Fuel Spring Model : Subsystem
  Disturbance Force : Outport
  Disturbance Moment : Outport  Port=2
  wires:
  Thrust/1 -> Fuel Spring Model/1(Thrust)
  Fuel Spring Model/1(Fuel Slosh Force) -> Disturbance Force/1
  Fuel Spring Model/2(Fuel Slosh Moment) -> Disturbance Moment/1

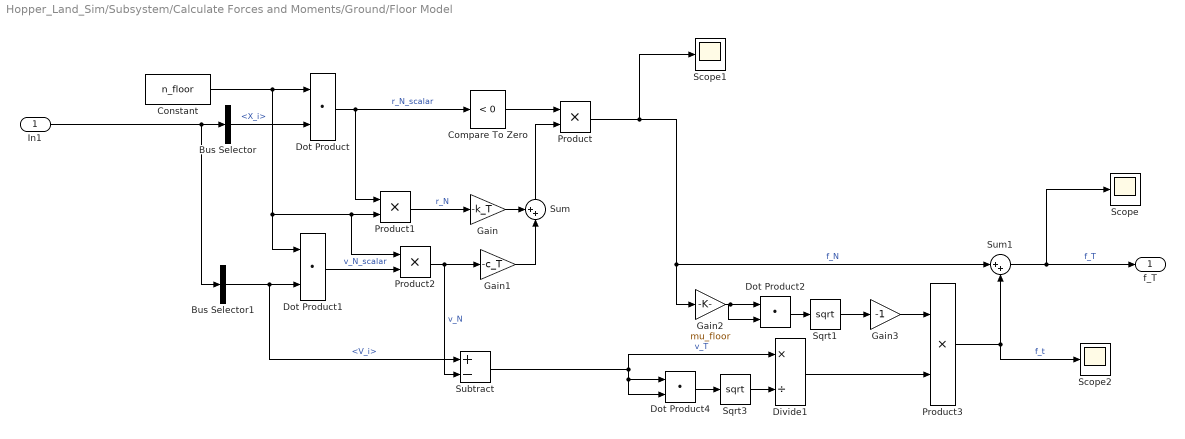
== system Hopper_Land_Sim/Subsystem/Calculate Forces and Moments/Ground/Floor Model ==
  In1 : Inport
  Bus Selector : BusSelector  OutputSignals=X_i
  Bus Selector1 : BusSelector  OutputSignals=V_i
  Compare To Zero : simulink/Logic and Bit Operations/Compare To Zero  relop=<  OutDataTypeStr=boolean
  Constant : Constant  Value=n_floor
  Divide1 : Product  Inputs=*/
  Dot Product{,1..2,4} (4 alike) : DotProduct  OutDataTypeStr=Inherit: Inherit via internal rule
  Gain : Gain  Gain=-k_T
  Gain1 : Gain  Gain=-c_T
  Gain2 : Gain  Gain=mu_floor
  Gain3 : Gain  Gain=-1
  Product{,1..3} (4 alike) : Product
  Scope : Scope
  Scope1 : Scope
  Scope2 : Scope
  Sqrt1 : Sqrt
  Sqrt3 : Sqrt
  Subtract : Sum  Inputs=+-
  Sum : Sum  Inputs=++|
  Sum1 : Sum  Inputs=|++
  f_T : Outport
  wires:
  Product2/1 -> Subtract/2, Gain1/1  "v_N"
  Bus Selector/1 -> Dot Product/2  "<X_i>"
  Constant/1 -> Dot Product1/1, Product2/1, Product1/2, Dot Product/1
  Bus Selector1/1 -> Subtract/1, Dot Product1/2  "<V_i>"
  Product3/1 -> Scope2/1, Sum1/2  "f_t"
  Dot Product1/1 -> Product2/2  "v_N_scalar"
  Product/1 -> Scope1/1, Gain2/1, Sum1/1  "f_N"
  Dot Product/1 -> Product1/1, Compare To Zero/1  "r_N_scalar"
  In1/1 -> Bus Selector1/1, Bus Selector/1
  Gain3/1 -> Product3/1
  Gain2/1 -> Dot Product2/2, Dot Product2/1
  Product1/1 -> Gain/1  "r_N"
  Sum1/1 -> f_T/1, Scope/1  "f_T"
  Dot Product2/1 -> Sqrt1/1
  Gain/1 -> Sum/1
  Sum/1 -> Product/2
  Compare To Zero/1 -> Product/1
  Gain1/1 -> Sum/2
  Sqrt1/1 -> Gain3/1
  Dot Product4/1 -> Sqrt3/1
  Divide1/1 -> Product3/2
  Sqrt3/1 -> Divide1/2
  Subtract/1 -> Divide1/1, Dot Product4/1, Dot Product4/2  "v_T"

== system Hopper_Land_Sim/Subsystem/Calculate Forces and Moments/Ground/Floor Model1 ==
  In1 : Inport
  Abs : Abs  SaturateOnIntegerOverflow=off
  Bus Selector : BusSelector  OutputSignals=X_i
  Compare To Zero : simulink/Logic and Bit Operations/Compare To Zero  relop=<  OutDataTypeStr=boolean
  Constant : Constant  Value=n_floor
  Constant1 : Constant  Value=[0; 0; 1000000]
  Dot Product : DotProduct  OutDataTypeStr=Inherit: Inherit via internal rule
  Product : Product
  f_T : Outport
  wires:
  Bus Selector/1 -> Dot Product/2  "<X_i>"
  Constant/1 -> Dot Product/1
  Dot Product/1 -> Compare To Zero/1  "r_N_scalar"
  In1/1 -> Bus Selector/1
  Compare To Zero/1 -> Product/1
  Product/1 -> Abs/1  "f_N"
  Abs/1 -> f_T/1
  Constant1/1 -> Product/2

== system Hopper_Land_Sim/Subsystem/Calculate Forces and Moments/Ground/Leg Model ==
  f_T : Inport
  Leg1 : Subsystem
  Leg2 : Subsystem
  Leg3 : Subsystem
  Leg4 : Subsystem
  Sum{1..2,5..6} (4 alike) : Sum  Inputs=++|
  Sum3 : Sum  Inputs=|++
  Sum4 : Sum  Inputs=|++
  Leg Force : Outport
  Leg Moment : Outport  Port=2
  wires:
  f_T/1 -> Leg4/1(f_T), Leg3/1(f_T), Leg2/1(f_T), Leg1/1(f_T)
  Leg3/1(f_l3) -> Sum1/1
  Leg4/1(f_l4) -> Sum1/2
  Leg2/1(f_l2) -> Sum2/1
  Sum1/1 -> Sum2/2
  ? -> Sum3/1
  Sum2/1 -> Sum3/2
  Leg1/1(m_l1) -> Sum4/1
  Leg2/2(m_l2) -> Sum5/1
  Leg3/2(m_l3) -> Sum6/1
  Leg4/2(m_l4) -> Sum6/2
  Sum6/1 -> Sum5/2
  Sum5/1 -> Sum4/2
  Sum3/1 -> Leg Force/1
  Sum4/1 -> Leg Moment/1

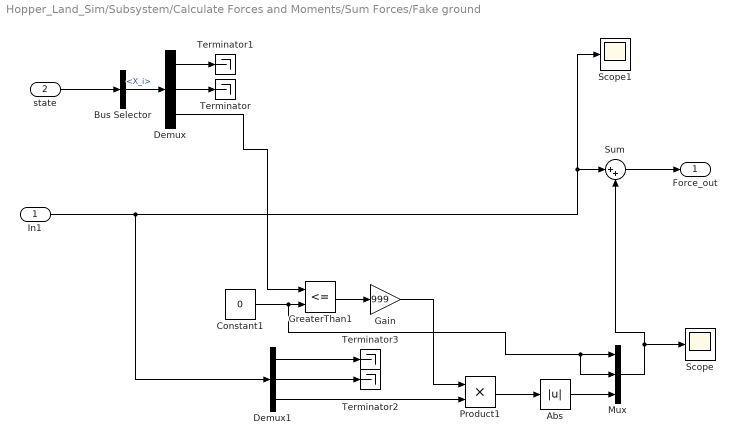
== system Hopper_Land_Sim/Subsystem/Calculate Forces and Moments/Sum Forces/Fake ground ==
  In1 : Inport
  state : Inport  Port=2
  Abs : Abs  SaturateOnIntegerOverflow=off
  Bus Selector : BusSelector  OutputSignals=X_i
  Constant1 : Constant  Value=0
  Demux : Demux  Outputs=3
  Demux1 : Demux  Outputs=3
  Gain : Gain  Gain=999
  GreaterThan1 : RelationalOperator  Operator=<=  OutDataTypeStr=boolean  RndMeth=Simplest  InputSameDT=off
  Mux : Mux  Inputs=3
  Product1 : Product
  Scope : Scope
  Scope1 : Scope
  Sum : Sum  Inputs=|++
  Terminator{,1..3} (4 alike) : Terminator
  Force_out : Outport
  wires:
  state/1 -> Bus Selector/1
  Bus Selector/1 -> Demux/1  "<X_i>"
  Demux/2 -> Terminator/1
  Demux/1 -> Terminator1/1
  Demux/3 -> GreaterThan1/1
  Constant1/1 -> Mux/2, Mux/1, GreaterThan1/2
  GreaterThan1/1 -> Gain/1
  Gain/1 -> Product1/1
  Product1/1 -> Abs/1
  Sum/1 -> Force_out/1
  In1/1 -> Demux1/1, Scope1/1, Sum/1
  Demux1/3 -> Product1/2
  Abs/1 -> Mux/3
  Demux1/2 -> Terminator2/1
  Demux1/1 -> Terminator3/1
  Mux/1 -> Sum/2, Scope/1

== system Hopper_Land_Sim/Subsystem/Calculate Forces and Moments/Sum Forces/Gravity ==
  state : Inport
  Bus Selector : BusSelector  OutputSignals=DCM_bi
  Constant1 : Constant  Value=[0; 0; -g]
  Gravity Force : Gain  Gain=m_e+m_l
  Matrix Multiply : Product  Multiplication=Matrix(*)
  gravity : Outport
  wires:
  Constant1/1 -> Matrix Multiply/2
  Gravity Force/1 -> gravity/1
  state/1 -> Bus Selector/1
  Bus Selector/1 -> Matrix Multiply/1  "<DCM_bi>"
  Matrix Multiply/1 -> Gravity Force/1

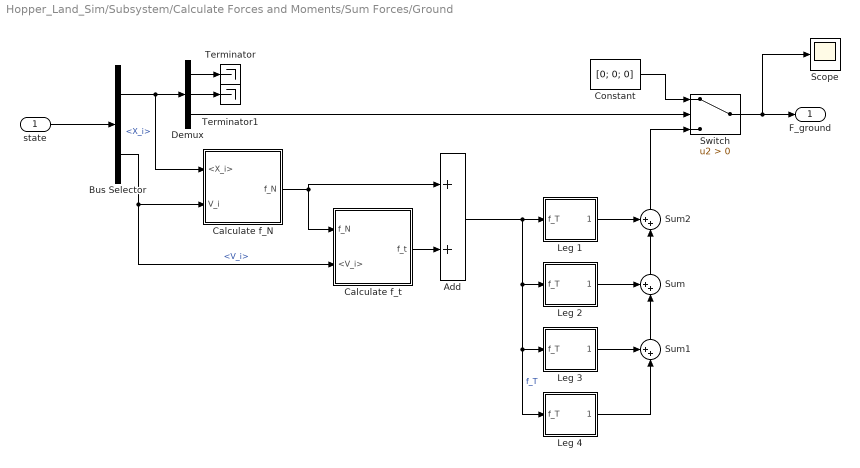
== system Hopper_Land_Sim/Subsystem/Calculate Forces and Moments/Sum Forces/Ground ==
  state : Inport
  Add : Sum
  Bus Selector : BusSelector  OutputSignals=X_i,V_i
  Calculate f_N : Subsystem
  Calculate f_t : Subsystem
  Constant : Constant  Value=[0; 0; 0]
  Demux : Demux  Outputs=3
  Leg 1 : Subsystem
  Leg 2 : Subsystem
  Leg 3 : Subsystem
  Leg 4 : Subsystem
  Scope : Scope
  Sum : Sum  Inputs=++|
  Sum1 : Sum  Inputs=++|
  Sum2 : Sum  Inputs=++|
  Switch : Switch  Criteria=u2 > Threshold  SaturateOnIntegerOverflow=off  InputSameDT=off
  Terminator : Terminator
  Terminator1 : Terminator
  F_ground : Outport
  wires:
  state/1 -> Bus Selector/1
  Bus Selector/1 -> Calculate f_N/1(<X_i>), Demux/1  "<X_i>"
  Demux/3 -> Switch/2
  Constant/1 -> Switch/1
  Switch/1 -> Scope/1, F_ground/1
  Bus Selector/2 -> Calculate f_t/2(<V_i>), Calculate f_N/2(V_i)  "<V_i>"
  Calculate f_N/1(f_N) -> Add/1, Calculate f_t/1(f_N)
  Calculate f_t/1(f_t) -> Add/2
  Add/1 -> Leg 1/1(f_T), Leg 2/1(f_T), Leg 4/1(f_T), Leg 3/1(f_T)  "f_T"
  Demux/1 -> Terminator/1
  Demux/2 -> Terminator1/1
  Leg 2/1(Outport) -> Sum/1
  Leg 3/1(Outport) -> Sum1/1
  Leg 4/1(Outport) -> Sum1/2
  Sum1/1 -> Sum/2
  Sum/1 -> Sum2/2
  Leg 1/1(Outport) -> Sum2/1
  Sum2/1 -> Switch/3

== system Hopper_Land_Sim/Subsystem/Calculate Forces and Moments/Disturbances/Fuel Slosh/Fuel Spring Model ==
  Thrust : Inport
  LOX Model : Subsystem
  Fuel Slosh Force : Outport
  Fuel Slosh Moment : Outport  Port=2
  wires:
  Thrust/1 -> LOX Model/1(Thrust)
  LOX Model/2(LOX Fuel Slosh Moment) -> Fuel Slosh Moment/1
  LOX Model/1(LOX Fuel Slosh Force) -> Fuel Slosh Force/1

== system Hopper_Land_Sim/Subsystem/Calculate Forces and Moments/Ground/Leg Model/Leg1 ==
  f_T : Inport
  Constant : Constant  Value=r_l1
  Cross Product : matrix_library/Cross Product
  Dot Product : DotProduct  OutDataTypeStr=Inherit: Inherit via internal rule
  Gain : Gain  Gain=1/m_s
  Gain1 : Gain
  Gain2 : Gain
  Integrator : Integrator
  Integrator1 : Integrator
  Product : Product
  Step : Step  Before=[0 0 100]  After=[0 0 0]  SampleTime=0
  Sum : Sum  Inputs=|++
  Sum1 : Sum  Inputs=|++
  m_l1 : Outport
  wires:
  f_T/1 -> Cross Product/1, Dot Product/1
  Constant/1 -> Cross Product/2, Product/2, Dot Product/2
  Dot Product/1 -> Product/1
  Product/1 -> ?  "f_Tt"
  ? -> m_l1/1
  Cross Product/1 -> ?  "f_Tn"
  Sum/1 -> Gain/1
  Integrator/1 -> Gain1/1, Integrator1/1  "d_dot*rhat"
  Integrator1/1 -> Gain2/1  "d"
  Sum1/1 -> Sum/2
  Step/1 -> Sum/1
  Gain/1 -> Integrator/1  "S_ddot"
  Gain1/1 -> Sum1/2
  Gain2/1 -> Sum1/1

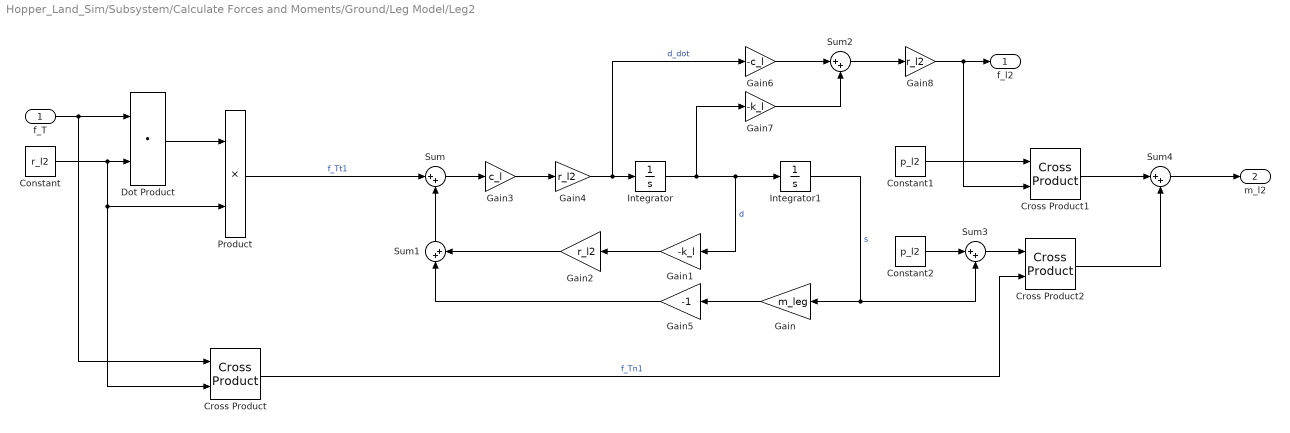
== system Hopper_Land_Sim/Subsystem/Calculate Forces and Moments/Ground/Leg Model/Leg2 ==
  f_T : Inport
  Constant : Constant  Value=r_l2
  Constant1 : Constant  Value=p_l2
  Constant2 : Constant  Value=p_l2
  Cross Product : matrix_library/Cross Product
  Cross Product1 : matrix_library/Cross Product
  Cross Product2 : matrix_library/Cross Product
  Dot Product : DotProduct  OutDataTypeStr=Inherit: Inherit via internal rule
  Gain : Gain  Gain=m_leg
  Gain1 : Gain  Gain=-k_l
  Gain2 : Gain  Gain=r_l2
  Gain3 : Gain  Gain=c_l
  Gain4 : Gain  Gain=r_l2
  Gain5 : Gain  Gain=-1
  Gain6 : Gain  Gain=-c_l
  Gain7 : Gain  Gain=-k_l
  Gain8 : Gain  Gain=r_l2
  Integrator : Integrator
  Integrator1 : Integrator
  Product : Product
  Sum{,1..4} (5 alike) : Sum  Inputs=|++
  f_l2 : Outport
  m_l2 : Outport  Port=2
  wires:
  Sum4/1 -> m_l2/1
  Cross Product2/1 -> Sum4/2
  Cross Product1/1 -> Sum4/1
  Sum3/1 -> Cross Product2/1
  Constant2/1 -> Sum3/1
  Constant1/1 -> Cross Product1/1
  Gain8/1 -> f_l2/1, Cross Product1/2
  Sum2/1 -> Gain8/1
  Gain7/1 -> Sum2/2
  Gain6/1 -> Sum2/1
  Gain5/1 -> Sum1/1
  Gain/1 -> Gain5/1
  Sum1/1 -> Sum/2
  Gain2/1 -> Sum1/2
  Sum/1 -> Gain3/1
  Gain4/1 -> Integrator/1, Gain6/1  "d_dot"
  Gain1/1 -> Gain2/1
  Integrator1/1 -> Gain/1, Sum3/2  "s"
  Integrator/1 -> Integrator1/1, Gain1/1, Gain7/1  "d"
  Gain3/1 -> Gain4/1
  Cross Product/1 -> Cross Product2/2  "f_Tn1"
  Product/1 -> Sum/1  "f_Tt1"
  Dot Product/1 -> Product/1
  Constant/1 -> Dot Product/2, Product/2, Cross Product/2
  f_T/1 -> Dot Product/1, Cross Product/1

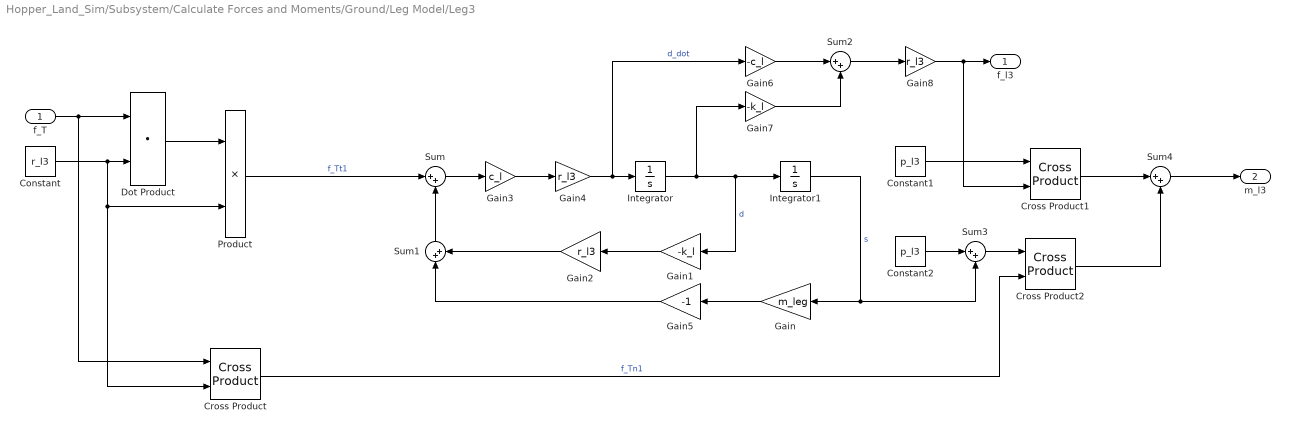
== system Hopper_Land_Sim/Subsystem/Calculate Forces and Moments/Ground/Leg Model/Leg3 ==
  f_T : Inport
  Constant : Constant  Value=r_l3
  Constant1 : Constant  Value=p_l3
  Constant2 : Constant  Value=p_l3
  Cross Product : matrix_library/Cross Product
  Cross Product1 : matrix_library/Cross Product
  Cross Product2 : matrix_library/Cross Product
  Dot Product : DotProduct  OutDataTypeStr=Inherit: Inherit via internal rule
  Gain : Gain  Gain=m_leg
  Gain1 : Gain  Gain=-k_l
  Gain2 : Gain  Gain=r_l3
  Gain3 : Gain  Gain=c_l
  Gain4 : Gain  Gain=r_l3
  Gain5 : Gain  Gain=-1
  Gain6 : Gain  Gain=-c_l
  Gain7 : Gain  Gain=-k_l
  Gain8 : Gain  Gain=r_l3
  Integrator : Integrator
  Integrator1 : Integrator
  Product : Product
  Sum{,1..4} (5 alike) : Sum  Inputs=|++
  f_l3 : Outport
  m_l3 : Outport  Port=2
  wires:
  f_T/1 -> Cross Product/1, Dot Product/1
  Constant/1 -> Cross Product/2, Product/2, Dot Product/2
  Dot Product/1 -> Product/1
  Product/1 -> Sum/1  "f_Tt1"
  Cross Product/1 -> Cross Product2/2  "f_Tn1"
  Gain3/1 -> Gain4/1
  Integrator/1 -> Gain7/1, Gain1/1, Integrator1/1  "d"
  Integrator1/1 -> Sum3/2, Gain/1  "s"
  Gain1/1 -> Gain2/1
  Gain4/1 -> Gain6/1, Integrator/1  "d_dot"
  Sum/1 -> Gain3/1
  Gain2/1 -> Sum1/2
  Sum1/1 -> Sum/2
  Gain/1 -> Gain5/1
  Gain5/1 -> Sum1/1
  Gain6/1 -> Sum2/1
  Gain7/1 -> Sum2/2
  Sum2/1 -> Gain8/1
  Gain8/1 -> Cross Product1/2, f_l3/1
  Constant1/1 -> Cross Product1/1
  Constant2/1 -> Sum3/1
  Sum3/1 -> Cross Product2/1
  Cross Product1/1 -> Sum4/1
  Cross Product2/1 -> Sum4/2
  Sum4/1 -> m_l3/1

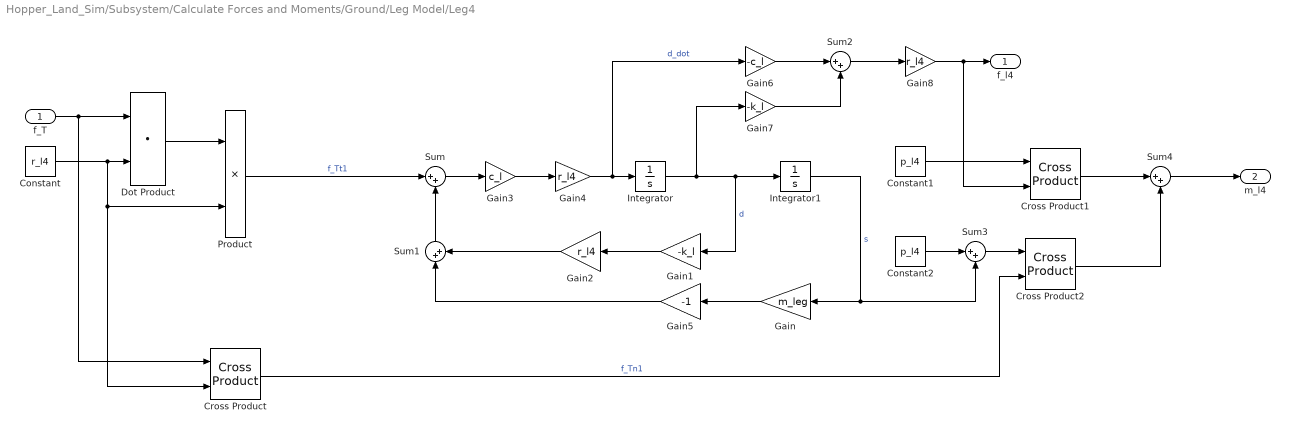
== system Hopper_Land_Sim/Subsystem/Calculate Forces and Moments/Ground/Leg Model/Leg4 ==
  f_T : Inport
  Constant : Constant  Value=r_l4
  Constant1 : Constant  Value=p_l4
  Constant2 : Constant  Value=p_l4
  Cross Product : matrix_library/Cross Product
  Cross Product1 : matrix_library/Cross Product
  Cross Product2 : matrix_library/Cross Product
  Dot Product : DotProduct  OutDataTypeStr=Inherit: Inherit via internal rule
  Gain : Gain  Gain=m_leg
  Gain1 : Gain  Gain=-k_l
  Gain2 : Gain  Gain=r_l4
  Gain3 : Gain  Gain=c_l
  Gain4 : Gain  Gain=r_l4
  Gain5 : Gain  Gain=-1
  Gain6 : Gain  Gain=-c_l
  Gain7 : Gain  Gain=-k_l
  Gain8 : Gain  Gain=r_l4
  Integrator : Integrator
  Integrator1 : Integrator
  Product : Product
  Sum{,1..4} (5 alike) : Sum  Inputs=|++
  f_l4 : Outport
  m_l4 : Outport  Port=2
  wires:
  Sum4/1 -> m_l4/1
  Cross Product2/1 -> Sum4/2
  Cross Product1/1 -> Sum4/1
  Sum3/1 -> Cross Product2/1
  Constant2/1 -> Sum3/1
  Constant1/1 -> Cross Product1/1
  Gain8/1 -> f_l4/1, Cross Product1/2
  Sum2/1 -> Gain8/1
  Gain7/1 -> Sum2/2
  Gain6/1 -> Sum2/1
  Gain5/1 -> Sum1/1
  Gain/1 -> Gain5/1
  Sum1/1 -> Sum/2
  Gain2/1 -> Sum1/2
  Sum/1 -> Gain3/1
  Gain4/1 -> Integrator/1, Gain6/1  "d_dot"
  Gain1/1 -> Gain2/1
  Integrator1/1 -> Gain/1, Sum3/2  "s"
  Integrator/1 -> Integrator1/1, Gain1/1, Gain7/1  "d"
  Gain3/1 -> Gain4/1
  Cross Product/1 -> Cross Product2/2  "f_Tn1"
  Product/1 -> Sum/1  "f_Tt1"
  Dot Product/1 -> Product/1
  Constant/1 -> Dot Product/2, Product/2, Cross Product/2
  f_T/1 -> Dot Product/1, Cross Product/1

== system Hopper_Land_Sim/Subsystem/Calculate Forces and Moments/Sum Forces/Ground/Calculate f_N ==
  <X_i> : Inport
  V_i : Inport  Port=2
  Add : Sum
  Constant : Constant  Value=n_surface
  Cross Product : matrix_library/Cross Product
  Gain : Gain  Gain=-k_T
  Gain1 : Gain  Gain=-C_T
  f_N : Outport
  wires:
  V_i/1 -> Cross Product/1
  Gain1/1 -> Add/2
  Gain/1 -> Add/1
  Add/1 -> f_N/1
  Constant/1 -> Cross Product/2
  Cross Product/1 -> Gain1/1
  <X_i>/1 -> Gain/1

== system Hopper_Land_Sim/Subsystem/Calculate Forces and Moments/Sum Forces/Ground/Calculate f_t ==
  f_N : Inport
  <V_i> : Inport  Port=2
  Abs : Abs  SaturateOnIntegerOverflow=off
  Constant : Constant  Value=n_surface
  Dot Product : DotProduct  OutDataTypeStr=Inherit: Inherit via internal rule
  Gain : Gain  Gain=mu_surface
  Gain1 : Gain  Gain=-1
  Normalize Vector : vrlib/Utilities/Normalize Vector  maxzero=0
  Product : Product
  f_t : Outport
  wires:
  f_N/1 -> Gain/1
  Constant/1 -> Dot Product/2
  <V_i>/1 -> Dot Product/1
  Dot Product/1 -> Normalize Vector/1  "v_T"
  Gain/1 -> Abs/1
  Normalize Vector/1 -> Product/2
  Abs/1 -> Product/1
  Product/1 -> Gain1/1
  Gain1/1 -> f_t/1

== system Hopper_Land_Sim/Subsystem/Calculate Forces and Moments/Sum Forces/Ground/Leg 1 ==
  f_T : Inport
  Constant : Constant  Value=r_l1
  Cross Product : matrix_library/Cross Product
  Dot Product : DotProduct  OutDataTypeStr=Inherit: Inherit via internal rule
  Product : Product
  Terminator : Terminator
  Outport : Outport
  wires:
  f_T/1 -> Cross Product/1, Dot Product/1
  Constant/1 -> Product/1, Cross Product/2, Dot Product/2
  Dot Product/1 -> Product/2
  Product/1 -> Outport/1  "F_Tt"
  Cross Product/1 -> Terminator/1  "F_Tn"

== system Hopper_Land_Sim/Subsystem/Calculate Forces and Moments/Sum Forces/Ground/Leg 2 ==
  f_T : Inport
  Constant : Constant  Value=r_l2
  Cross Product : matrix_library/Cross Product
  Dot Product : DotProduct  OutDataTypeStr=Inherit: Inherit via internal rule
  Product : Product
  Terminator : Terminator
  Outport : Outport
  wires:
  Cross Product/1 -> Terminator/1  "F_Tn"
  Product/1 -> Outport/1  "F_Tt"
  Dot Product/1 -> Product/2
  Constant/1 -> Dot Product/2, Cross Product/2
  f_T/1 -> Product/1, Dot Product/1, Cross Product/1

== system Hopper_Land_Sim/Subsystem/Calculate Forces and Moments/Sum Forces/Ground/Leg 3 ==
  f_T : Inport
  Constant : Constant  Value=r_l3
  Cross Product : matrix_library/Cross Product
  Dot Product : DotProduct  OutDataTypeStr=Inherit: Inherit via internal rule
  Product : Product
  Terminator : Terminator
  Outport : Outport
  wires:
  f_T/1 -> Cross Product/1, Dot Product/1, Product/1
  Constant/1 -> Cross Product/2, Dot Product/2
  Dot Product/1 -> Product/2
  Product/1 -> Outport/1  "F_Tt"
  Cross Product/1 -> Terminator/1  "F_Tn"

== system Hopper_Land_Sim/Subsystem/Calculate Forces and Moments/Sum Forces/Ground/Leg 4 ==
  f_T : Inport
  Constant : Constant  Value=r_l4
  Cross Product : matrix_library/Cross Product
  Dot Product : DotProduct  OutDataTypeStr=Inherit: Inherit via internal rule
  Product : Product
  Terminator : Terminator
  Outport : Outport
  wires:
  Cross Product/1 -> Terminator/1  "F_Tn"
  Product/1 -> Outport/1  "F_Tt"
  Dot Product/1 -> Product/2
  Constant/1 -> Dot Product/2, Cross Product/2
  f_T/1 -> Product/1, Dot Product/1, Cross Product/1

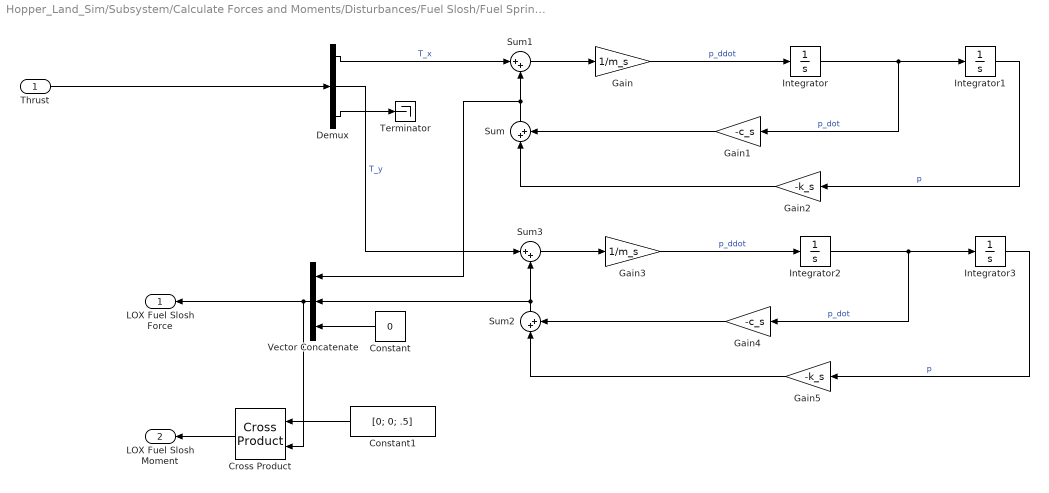
== system Hopper_Land_Sim/Subsystem/Calculate Forces and Moments/Disturbances/Fuel Slosh/Fuel Spring Model/LOX Model ==
  Thrust : Inport
  Constant : Constant  Value=0
  Constant1 : Constant  Value=[0; 0; .5]
  Cross Product : matrix_library/Cross Product
  Demux : Demux  Outputs=3
  Gain : Gain  Gain=1/m_s
  Gain1 : Gain  Gain=-c_s
  Gain2 : Gain  Gain=-k_s
  Gain3 : Gain  Gain=1/m_s
  Gain4 : Gain  Gain=-c_s
  Gain5 : Gain  Gain=-k_s
  Integrator{,1..3} (4 alike) : Integrator
  Sum{,1..3} (4 alike) : Sum  Inputs=|++
  Terminator : Terminator
  Vector Concatenate : Concatenate  NumInputs=3
  LOX Fuel Slosh Force : Outport
  LOX Fuel Slosh Moment : Outport  Port=2
  wires:
  Sum/1 -> Vector Concatenate/1, Sum1/2
  Gain4/1 -> Sum2/2
  Gain2/1 -> Sum/1
  Integrator2/1 -> Gain4/1, Integrator3/1  "p_dot"
  Demux/2 -> Sum3/1  "T_y"
  Sum2/1 -> Sum3/2, Vector Concatenate/2
  Constant1/1 -> Cross Product/1
  Sum3/1 -> Gain3/1
  Integrator/1 -> Gain1/1, Integrator1/1  "p_dot"
  Gain5/1 -> Sum2/1
  Constant/1 -> Vector Concatenate/3
  Demux/1 -> Sum1/1  "T_x"
  Gain3/1 -> Integrator2/1  "p_ddot"
  Integrator1/1 -> Gain2/1  "p"
  Cross Product/1 -> LOX Fuel Slosh Moment/1
  Gain1/1 -> Sum/2
  Vector Concatenate/1 -> LOX Fuel Slosh Force/1, Cross Product/2
  Sum1/1 -> Gain/1
  Integrator3/1 -> Gain5/1  "p"
  Gain/1 -> Integrator/1  "p_ddot"
  Demux/3 -> Terminator/1
  Thrust/1 -> Demux/1

== matlab function Hopper_Land_Sim/Controller/X-Y control/junk/Calculate LQR Gains (X-Theta) ==
  data: State input; K output
function K = IterativeLQR(State)
K = IterativeLQR(State);
end

== matlab function Hopper_Land_Sim/Controller/pqr to theta_dot/MATLAB Function ==
  data: euler_a_rad input; euler_dot output; omega_b input
function euler_dot = EulerRates(euler_a_rad, omega_b)
p = omega_b(1);
q = omega_b(2);
r = omega_b(3);

phi = euler_a_rad(1);
theta = euler_a_rad(2);
psi = euler_a_rad(3);

euler_dot = [p + (q*sin(phi) + r*cos(phi))*tan(theta);
             q*cos(phi) - r*sin(phi);
             (q*sin(phi) +r*cos(phi))/cos(theta)];

== matlab function Hopper_Land_Sim/Controller/X-Y control/junk/Calculate LQR Gains (Y-Phi) ==
  data: State input; K output
function K = IterativeLQR(State)
K = IterativeLQR(State);
end
